simulink library "HighClearance_library"  (R2019b)
settings: Solver=VariableStepAuto  StartTime=0.0  StopTime=10.0  RelTol=1e-3
undefined symbols (not defined in the file): bangBang_maxOut, baseClearance, controlTolerance, controlWaitTime, ctrlWarningTime, currentControl_IC, currentControl_Ki, currentControl_Kp, currentControl_maxOut, currentControl_minOut, defaultPositionSensor_BrkPnts, DiscIntNeverNeededParam, errDelay, heightCalibrating_e, heightControlToleranceStart, heightControlToleranceStop, heightDiffTolerance, heightDown_e, heightError_e, heightMovingDown_e, heightMovingUp_e, heightTolerance, heightToleranceRoad, heightUnknown_e, heightUp_e, IOD_OK, legMovingTimeout, minDistanceMoving, movementTimeOut, noMovementTimeOut, plausiDistance, positionControl_IC, positionControl_Ki, positionControl_Kp, positionControl_maxOut, positionControl_minOut, positionSensor_tblData, sensorCutOffHz, step_time, trackWidthTolerance, useSensorFilter
libraries: $bdroot x29, simulink x1
settings Model: Creator=lemaya  LastModifiedBy=milesluc
settings DataIOCC: ReturnWorkspaceOutputs=off
settings DebuggingCC: ArithmeticOperatorsInVariantConditions=warning
settings SFSimCC: SimUseLocalCustomCode=off  CustomCodeUndefinedFunction=UseInterfaceOnly
settings RTWCC: RTWUseLocalCustomCode=off
settings CodeAppCC: StateflowObjectComments=on

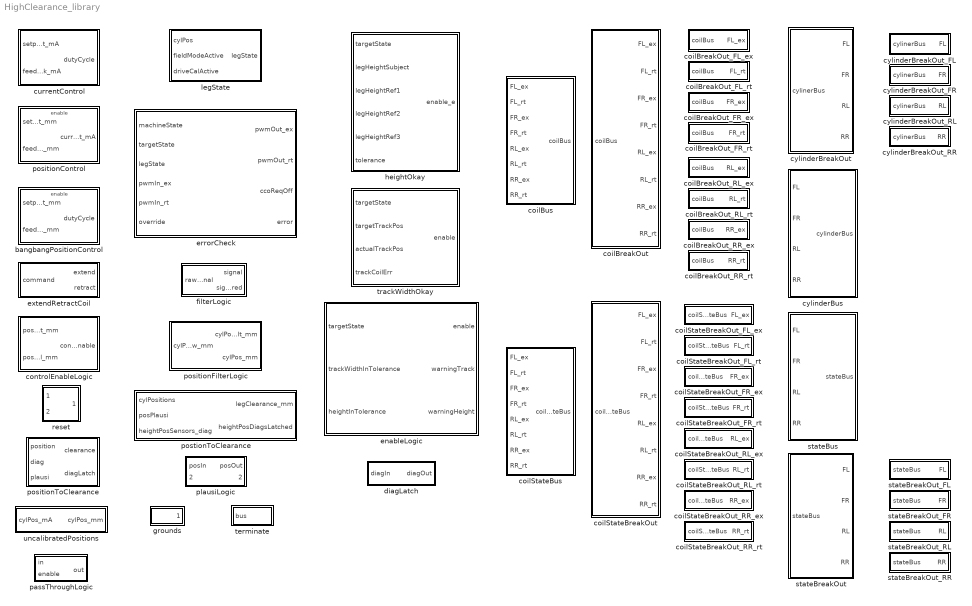
== system HighClearance_library ==
  bangbangPositionControl : Subsystem
  coilBreakOut : Subsystem
  coilBreakOut_FL_ex : Subsystem
  coilBreakOut_FL_rt : Subsystem
  coilBreakOut_FR_ex : Subsystem
  coilBreakOut_FR_rt : Subsystem
  coilBreakOut_RL_ex : Subsystem
  coilBreakOut_RL_rt : Subsystem
  coilBreakOut_RR_ex : Subsystem
  coilBreakOut_RR_rt : Subsystem
  coilBus : Subsystem
  coilStateBreakOut : Subsystem
  coilStateBreakOut_FL_ex : Subsystem
  coilStateBreakOut_FL_rt : Subsystem
  coilStateBreakOut_FR_ex : Subsystem
  coilStateBreakOut_FR_rt : Subsystem
  coilStateBreakOut_RL_ex : Subsystem
  coilStateBreakOut_RL_rt : Subsystem
  coilStateBreakOut_RR_ex : Subsystem
  coilStateBreakOut_RR_rt : Subsystem
  coilStateBus : Subsystem
  controlEnableLogic : Subsystem
  currentControl : Subsystem
  cylinderBreakOut : Subsystem
  cylinderBreakOut_FL : Subsystem
  cylinderBreakOut_FR : Subsystem
  cylinderBreakOut_RL : Subsystem
  cylinderBreakOut_RR : Subsystem
  cylinderBus : Subsystem
  diagLatch : Stateflow chart  TreatAsAtomicUnit=on
  enableLogic : Stateflow chart  TreatAsAtomicUnit=on
  errorCheck : Stateflow chart  TreatAsAtomicUnit=on
  extendRetractCoil : Subsystem
  filterLogic : Subsystem
  grounds : Subsystem
  heightOkay : Stateflow chart  TreatAsAtomicUnit=on
  legState : Stateflow chart  TreatAsAtomicUnit=on
  passThroughLogic : Subsystem
  plausiLogic : Subsystem
  positionControl : Subsystem
  positionFilterLogic : Subsystem
  positionToClearance : Subsystem
  postionToClearance : Subsystem
  reset : Subsystem
  stateBreakOut : Subsystem
  stateBreakOut_FL : Subsystem
  stateBreakOut_FR : Subsystem
  stateBreakOut_RL : Subsystem
  stateBreakOut_RR : Subsystem
  stateBus : Subsystem
  terminate : Subsystem
  trackWidthOkay : Stateflow chart  TreatAsAtomicUnit=on
  uncalibratedPositions : Subsystem

== system HighClearance_library/bangbangPositionControl ==
  setpoint_mm : Inport
  feedback_mm : Inport  Port=2
  Enable : EnablePort  StatesWhenEnabling=reset
  Sum : Sum  Inputs=|+-
  extendRetractLogic : Stateflow chart  TreatAsAtomicUnit=on
  dutyCycle : Outport  OutputWhenDisabled=reset  InitialOutput=[0]
  wires:
  extendRetractLogic/1(pwm) -> dutyCycle/1
  Sum/1 -> extendRetractLogic/1(error)
  feedback_mm/1 -> Sum/2
  setpoint_mm/1 -> Sum/1

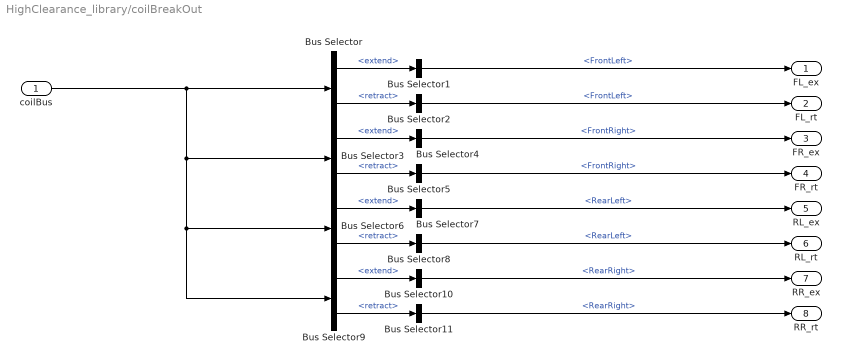
== system HighClearance_library/coilBreakOut ==
  coilBus : Inport  OutDataTypeStr=Bus: CoilBus
  Bus Selector{,3,6,9} (4 alike) : BusSelector  OutputSignals=extend,retract
  Bus Selector1 : BusSelector  OutputSignals=FrontLeft
  Bus Selector10 : BusSelector  OutputSignals=RearRight
  Bus Selector11 : BusSelector  OutputSignals=RearRight
  Bus Selector2 : BusSelector  OutputSignals=FrontLeft
  Bus Selector4 : BusSelector  OutputSignals=FrontRight
  Bus Selector5 : BusSelector  OutputSignals=FrontRight
  Bus Selector7 : BusSelector  OutputSignals=RearLeft
  Bus Selector8 : BusSelector  OutputSignals=RearLeft
  FL_ex : Outport
  FL_rt : Outport  Port=2
  FR_ex : Outport  Port=3
  FR_rt : Outport  Port=4
  RL_ex : Outport  Port=5
  RL_rt : Outport  Port=6
  RR_ex : Outport  Port=7
  RR_rt : Outport  Port=8
  wires:
  coilBus/1 -> Bus Selector/1, Bus Selector3/1, Bus Selector6/1, Bus Selector9/1
  Bus Selector9/2 -> Bus Selector11/1  "<retract>"
  Bus Selector11/1 -> RR_rt/1  "<RearRight>"
  Bus Selector10/1 -> RR_ex/1  "<RearRight>"
  Bus Selector9/1 -> Bus Selector10/1  "<extend>"
  Bus Selector6/2 -> Bus Selector8/1  "<retract>"
  Bus Selector8/1 -> RL_rt/1  "<RearLeft>"
  Bus Selector7/1 -> RL_ex/1  "<RearLeft>"
  Bus Selector6/1 -> Bus Selector7/1  "<extend>"
  Bus Selector3/2 -> Bus Selector5/1  "<retract>"
  Bus Selector5/1 -> FR_rt/1  "<FrontRight>"
  Bus Selector4/1 -> FR_ex/1  "<FrontRight>"
  Bus Selector3/1 -> Bus Selector4/1  "<extend>"
  Bus Selector/2 -> Bus Selector2/1  "<retract>"
  Bus Selector2/1 -> FL_rt/1  "<FrontLeft>"
  Bus Selector1/1 -> FL_ex/1  "<FrontLeft>"
  Bus Selector/1 -> Bus Selector1/1  "<extend>"

== system HighClearance_library/coilBreakOut_FL_ex ==
  coilBus : Inport  OutDataTypeStr=Bus: CoilBus
  Bus Selector : BusSelector  OutputSignals=extend
  Bus Selector1 : BusSelector  OutputSignals=FrontLeft
  FL_ex : Outport
  wires:
  Bus Selector/1 -> Bus Selector1/1  "<extend>"
  Bus Selector1/1 -> FL_ex/1  "<FrontLeft>"
  coilBus/1 -> Bus Selector/1

== system HighClearance_library/coilBreakOut_FL_rt ==
  coilBus : Inport  OutDataTypeStr=Bus: CoilBus
  Bus Selector : BusSelector  OutputSignals=retract
  Bus Selector1 : BusSelector  OutputSignals=FrontLeft
  FL_rt : Outport
  wires:
  coilBus/1 -> Bus Selector/1
  Bus Selector1/1 -> FL_rt/1  "<FrontLeft>"
  Bus Selector/1 -> Bus Selector1/1  "<retract>"

== system HighClearance_library/coilBreakOut_FR_ex ==
  coilBus : Inport  OutDataTypeStr=Bus: CoilBus
  Bus Selector : BusSelector  OutputSignals=extend
  Bus Selector1 : BusSelector  OutputSignals=FrontRight
  FR_ex : Outport
  wires:
  coilBus/1 -> Bus Selector/1
  Bus Selector1/1 -> FR_ex/1  "<FrontRight>"
  Bus Selector/1 -> Bus Selector1/1  "<extend>"

== system HighClearance_library/coilBreakOut_FR_rt ==
  coilBus : Inport  OutDataTypeStr=Bus: CoilBus
  Bus Selector : BusSelector  OutputSignals=retract
  Bus Selector1 : BusSelector  OutputSignals=FrontRight
  FR_rt : Outport
  wires:
  Bus Selector/1 -> Bus Selector1/1  "<retract>"
  Bus Selector1/1 -> FR_rt/1  "<FrontRight>"
  coilBus/1 -> Bus Selector/1

== system HighClearance_library/coilBreakOut_RL_ex ==
  coilBus : Inport  OutDataTypeStr=Bus: CoilBus
  Bus Selector : BusSelector  OutputSignals=extend
  Bus Selector1 : BusSelector  OutputSignals=RearLeft
  RL_ex : Outport
  wires:
  coilBus/1 -> Bus Selector/1
  Bus Selector1/1 -> RL_ex/1  "<RearLeft>"
  Bus Selector/1 -> Bus Selector1/1  "<extend>"

== system HighClearance_library/coilBreakOut_RL_rt ==
  coilBus : Inport  OutDataTypeStr=Bus: CoilBus
  Bus Selector : BusSelector  OutputSignals=retract
  Bus Selector1 : BusSelector  OutputSignals=RearLeft
  RL_rt : Outport
  wires:
  Bus Selector/1 -> Bus Selector1/1  "<retract>"
  Bus Selector1/1 -> RL_rt/1  "<RearLeft>"
  coilBus/1 -> Bus Selector/1

== system HighClearance_library/coilBreakOut_RR_ex ==
  coilBus : Inport  OutDataTypeStr=Bus: CoilBus
  Bus Selector : BusSelector  OutputSignals=extend
  Bus Selector1 : BusSelector  OutputSignals=RearRight
  RR_ex : Outport
  wires:
  Bus Selector/1 -> Bus Selector1/1  "<extend>"
  Bus Selector1/1 -> RR_ex/1  "<RearRight>"
  coilBus/1 -> Bus Selector/1

== system HighClearance_library/coilBreakOut_RR_rt ==
  coilBus : Inport  OutDataTypeStr=Bus: CoilBus
  Bus Selector : BusSelector  OutputSignals=retract
  Bus Selector1 : BusSelector  OutputSignals=RearRight
  RR_rt : Outport
  wires:
  coilBus/1 -> Bus Selector/1
  Bus Selector1/1 -> RR_rt/1  "<RearRight>"
  Bus Selector/1 -> Bus Selector1/1  "<retract>"

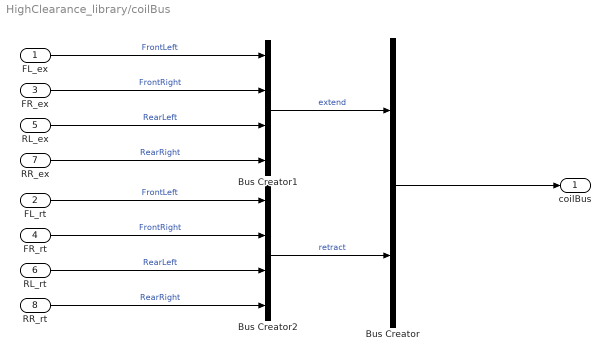
== system HighClearance_library/coilBus ==
  FL_ex : Inport
  FL_rt : Inport  Port=2
  FR_ex : Inport  Port=3
  FR_rt : Inport  Port=4
  RL_ex : Inport  Port=5
  RL_rt : Inport  Port=6
  RR_ex : Inport  Port=7
  RR_rt : Inport  Port=8
  Bus Creator : BusCreator  Inputs=2  OutDataTypeStr=Bus: CoilBus  NonVirtualBus=on
  Bus Creator1 : BusCreator  Inputs=4  OutDataTypeStr=Bus: CylinderBus  NonVirtualBus=on
  Bus Creator2 : BusCreator  Inputs=4  OutDataTypeStr=Bus: CylinderBus  NonVirtualBus=on
  coilBus : Outport  OutDataTypeStr=Bus: CoilBus
  wires:
  FL_ex/1 -> Bus Creator1/1  "FrontLeft"
  Bus Creator/1 -> coilBus/1
  FR_ex/1 -> Bus Creator1/2  "FrontRight"
  RL_ex/1 -> Bus Creator1/3  "RearLeft"
  RR_ex/1 -> Bus Creator1/4  "RearRight"
  Bus Creator1/1 -> Bus Creator/1  "extend"
  Bus Creator2/1 -> Bus Creator/2  "retract"
  FL_rt/1 -> Bus Creator2/1  "FrontLeft"
  FR_rt/1 -> Bus Creator2/2  "FrontRight"
  RL_rt/1 -> Bus Creator2/3  "RearLeft"
  RR_rt/1 -> Bus Creator2/4  "RearRight"

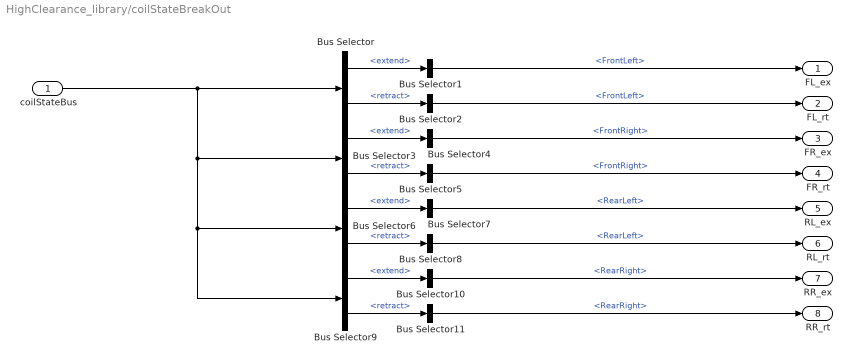
== system HighClearance_library/coilStateBreakOut ==
  coilStateBus : Inport  OutDataTypeStr=Bus: CoilStateBus
  Bus Selector{,3,6,9} (4 alike) : BusSelector  OutputSignals=extend,retract
  Bus Selector1 : BusSelector  OutputSignals=FrontLeft
  Bus Selector10 : BusSelector  OutputSignals=RearRight
  Bus Selector11 : BusSelector  OutputSignals=RearRight
  Bus Selector2 : BusSelector  OutputSignals=FrontLeft
  Bus Selector4 : BusSelector  OutputSignals=FrontRight
  Bus Selector5 : BusSelector  OutputSignals=FrontRight
  Bus Selector7 : BusSelector  OutputSignals=RearLeft
  Bus Selector8 : BusSelector  OutputSignals=RearLeft
  FL_ex : Outport
  FL_rt : Outport  Port=2
  FR_ex : Outport  Port=3
  FR_rt : Outport  Port=4
  RL_ex : Outport  Port=5
  RL_rt : Outport  Port=6
  RR_ex : Outport  Port=7
  RR_rt : Outport  Port=8
  wires:
  coilStateBus/1 -> Bus Selector/1, Bus Selector3/1, Bus Selector6/1, Bus Selector9/1
  Bus Selector9/2 -> Bus Selector11/1  "<retract>"
  Bus Selector11/1 -> RR_rt/1  "<RearRight>"
  Bus Selector10/1 -> RR_ex/1  "<RearRight>"
  Bus Selector9/1 -> Bus Selector10/1  "<extend>"
  Bus Selector6/2 -> Bus Selector8/1  "<retract>"
  Bus Selector8/1 -> RL_rt/1  "<RearLeft>"
  Bus Selector7/1 -> RL_ex/1  "<RearLeft>"
  Bus Selector6/1 -> Bus Selector7/1  "<extend>"
  Bus Selector3/2 -> Bus Selector5/1  "<retract>"
  Bus Selector5/1 -> FR_rt/1  "<FrontRight>"
  Bus Selector4/1 -> FR_ex/1  "<FrontRight>"
  Bus Selector3/1 -> Bus Selector4/1  "<extend>"
  Bus Selector/2 -> Bus Selector2/1  "<retract>"
  Bus Selector2/1 -> FL_rt/1  "<FrontLeft>"
  Bus Selector1/1 -> FL_ex/1  "<FrontLeft>"
  Bus Selector/1 -> Bus Selector1/1  "<extend>"

== system HighClearance_library/coilStateBreakOut_FL_ex ==
  coilStateBus : Inport  OutDataTypeStr=Bus: CoilStateBus
  Bus Selector : BusSelector  OutputSignals=extend
  Bus Selector1 : BusSelector  OutputSignals=FrontLeft
  FL_ex : Outport
  wires:
  Bus Selector/1 -> Bus Selector1/1  "<extend>"
  Bus Selector1/1 -> FL_ex/1  "<FrontLeft>"
  coilStateBus/1 -> Bus Selector/1

== system HighClearance_library/coilStateBreakOut_FL_rt ==
  coilStateBus : Inport  OutDataTypeStr=Bus: CoilStateBus
  Bus Selector : BusSelector  OutputSignals=retract
  Bus Selector1 : BusSelector  OutputSignals=FrontLeft
  FL_rt : Outport
  wires:
  coilStateBus/1 -> Bus Selector/1
  Bus Selector1/1 -> FL_rt/1  "<FrontLeft>"
  Bus Selector/1 -> Bus Selector1/1  "<retract>"

== system HighClearance_library/coilStateBreakOut_FR_ex ==
  coilStateBus : Inport  OutDataTypeStr=Bus: CoilStateBus
  Bus Selector : BusSelector  OutputSignals=extend
  Bus Selector1 : BusSelector  OutputSignals=FrontRight
  FR_ex : Outport
  wires:
  coilStateBus/1 -> Bus Selector/1
  Bus Selector1/1 -> FR_ex/1  "<FrontRight>"
  Bus Selector/1 -> Bus Selector1/1  "<extend>"

== system HighClearance_library/coilStateBreakOut_FR_rt ==
  coilStateBus : Inport  OutDataTypeStr=Bus: CoilStateBus
  Bus Selector : BusSelector  OutputSignals=retract
  Bus Selector1 : BusSelector  OutputSignals=FrontRight
  FR_rt : Outport
  wires:
  Bus Selector/1 -> Bus Selector1/1  "<retract>"
  Bus Selector1/1 -> FR_rt/1  "<FrontRight>"
  coilStateBus/1 -> Bus Selector/1

== system HighClearance_library/coilStateBreakOut_RL_ex ==
  coilStateBus : Inport  OutDataTypeStr=Bus: CoilStateBus
  Bus Selector : BusSelector  OutputSignals=extend
  Bus Selector1 : BusSelector  OutputSignals=RearLeft
  RL_ex : Outport
  wires:
  coilStateBus/1 -> Bus Selector/1
  Bus Selector1/1 -> RL_ex/1  "<RearLeft>"
  Bus Selector/1 -> Bus Selector1/1  "<extend>"

== system HighClearance_library/coilStateBreakOut_RL_rt ==
  coilStateBus : Inport  OutDataTypeStr=Bus: CoilStateBus
  Bus Selector : BusSelector  OutputSignals=retract
  Bus Selector1 : BusSelector  OutputSignals=RearLeft
  RL_rt : Outport
  wires:
  Bus Selector/1 -> Bus Selector1/1  "<retract>"
  Bus Selector1/1 -> RL_rt/1  "<RearLeft>"
  coilStateBus/1 -> Bus Selector/1

== system HighClearance_library/coilStateBreakOut_RR_ex ==
  coilStateBus : Inport  OutDataTypeStr=Bus: CoilStateBus
  Bus Selector : BusSelector  OutputSignals=extend
  Bus Selector1 : BusSelector  OutputSignals=RearRight
  RR_ex : Outport
  wires:
  Bus Selector/1 -> Bus Selector1/1  "<extend>"
  Bus Selector1/1 -> RR_ex/1  "<RearRight>"
  coilStateBus/1 -> Bus Selector/1

== system HighClearance_library/coilStateBreakOut_RR_rt ==
  coilStateBus : Inport  OutDataTypeStr=Bus: CoilStateBus
  Bus Selector : BusSelector  OutputSignals=retract
  Bus Selector1 : BusSelector  OutputSignals=RearRight
  RR_rt : Outport
  wires:
  coilStateBus/1 -> Bus Selector/1
  Bus Selector1/1 -> RR_rt/1  "<RearRight>"
  Bus Selector/1 -> Bus Selector1/1  "<retract>"

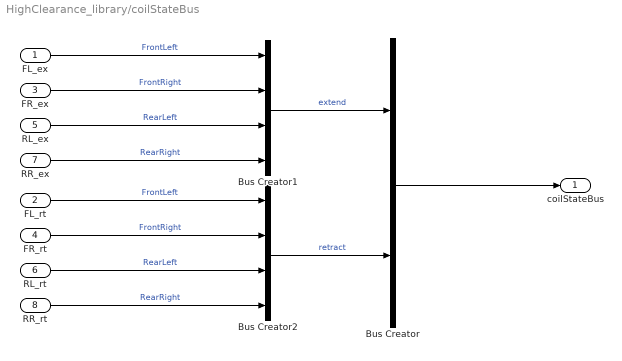
== system HighClearance_library/coilStateBus ==
  FL_ex : Inport
  FL_rt : Inport  Port=2
  FR_ex : Inport  Port=3
  FR_rt : Inport  Port=4
  RL_ex : Inport  Port=5
  RL_rt : Inport  Port=6
  RR_ex : Inport  Port=7
  RR_rt : Inport  Port=8
  Bus Creator : BusCreator  Inputs=2  OutDataTypeStr=Bus: CoilStateBus
  Bus Creator1 : BusCreator  Inputs=4  OutDataTypeStr=Bus: StateBus
  Bus Creator2 : BusCreator  Inputs=4  OutDataTypeStr=Bus: StateBus
  coilStateBus : Outport  OutDataTypeStr=Bus: CoilStateBus
  wires:
  FL_ex/1 -> Bus Creator1/1  "FrontLeft"
  Bus Creator/1 -> coilStateBus/1
  FR_ex/1 -> Bus Creator1/2  "FrontRight"
  RL_ex/1 -> Bus Creator1/3  "RearLeft"
  RR_ex/1 -> Bus Creator1/4  "RearRight"
  Bus Creator1/1 -> Bus Creator/1  "extend"
  Bus Creator2/1 -> Bus Creator/2  "retract"
  FL_rt/1 -> Bus Creator2/1  "FrontLeft"
  FR_rt/1 -> Bus Creator2/2  "FrontRight"
  RL_rt/1 -> Bus Creator2/3  "RearLeft"
  RR_rt/1 -> Bus Creator2/4  "RearRight"

== system HighClearance_library/controlEnableLogic ==
  postionTarget_mm : Inport
  positionActual_mm : Inport  Port=2
  enableLogic : Stateflow chart  TreatAsAtomicUnit=on
  controlEnable : Outport
  wires:
  postionTarget_mm/1 -> enableLogic/1(target)
  positionActual_mm/1 -> enableLogic/2(position)
  enableLogic/1(enable) -> controlEnable/1

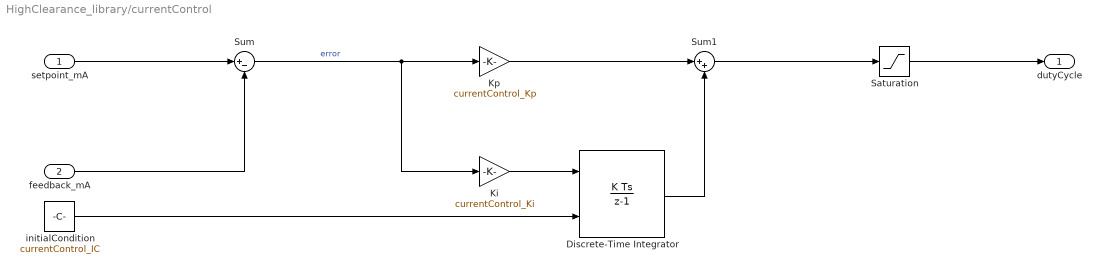
== system HighClearance_library/currentControl ==
  setpoint_mA : Inport
  feedback_mA : Inport  Port=2
  Discrete-Time Integrator : DiscreteIntegrator  InitialConditionSource=external  SampleTime=step_time  LimitOutput=on  UpperSaturationLimit=currentControl_maxOut  LowerSaturationLimit=currentControl_minOut  ICPrevOutput=DiscIntNeverNeededParam  ICPrevScaledInput=DiscIntNeverNeededParam
  Ki : Gain  Gain=currentControl_Ki
  Kp : Gain  Gain=currentControl_Kp
  Saturation : Saturate  UpperLimit=currentControl_maxOut  LowerLimit=currentControl_minOut
  Sum : Sum  Inputs=|+-
  Sum1 : Sum  Inputs=|++
  initialCondition : Constant  Value=currentControl_IC
  dutyCycle : Outport
  wires:
  Saturation/1 -> dutyCycle/1
  initialCondition/1 -> Discrete-Time Integrator/2
  Sum1/1 -> Saturation/1
  Discrete-Time Integrator/1 -> Sum1/2
  Ki/1 -> Discrete-Time Integrator/1
  Kp/1 -> Sum1/1
  Sum/1 -> Kp/1, Ki/1  "error"
  feedback_mA/1 -> Sum/2
  setpoint_mA/1 -> Sum/1

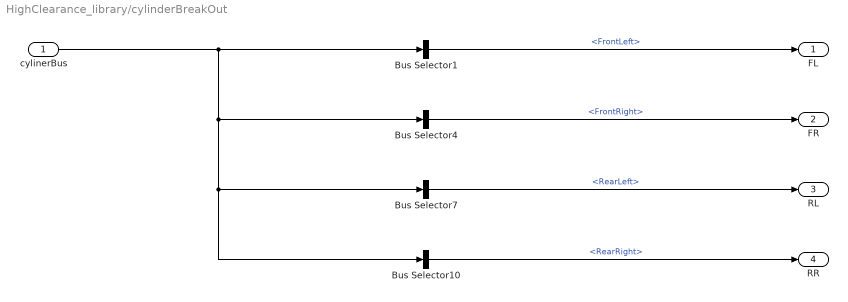
== system HighClearance_library/cylinderBreakOut ==
  cylinerBus : Inport  OutDataTypeStr=Bus: CylinderBus
  Bus Selector1 : BusSelector  OutputSignals=FrontLeft
  Bus Selector10 : BusSelector  OutputSignals=RearRight
  Bus Selector4 : BusSelector  OutputSignals=FrontRight
  Bus Selector7 : BusSelector  OutputSignals=RearLeft
  FL : Outport
  FR : Outport  Port=2
  RL : Outport  Port=3
  RR : Outport  Port=4
  wires:
  cylinerBus/1 -> Bus Selector1/1, Bus Selector4/1, Bus Selector7/1, Bus Selector10/1
  Bus Selector10/1 -> RR/1  "<RearRight>"
  Bus Selector7/1 -> RL/1  "<RearLeft>"
  Bus Selector4/1 -> FR/1  "<FrontRight>"
  Bus Selector1/1 -> FL/1  "<FrontLeft>"

== system HighClearance_library/cylinderBreakOut_FL ==
  cylinerBus : Inport  OutDataTypeStr=Bus: CylinderBus
  Bus Selector1 : BusSelector  OutputSignals=FrontLeft
  FL : Outport
  wires:
  cylinerBus/1 -> Bus Selector1/1
  Bus Selector1/1 -> FL/1  "<FrontLeft>"

== system HighClearance_library/cylinderBreakOut_FR ==
  cylinerBus : Inport  OutDataTypeStr=Bus: CylinderBus
  Bus Selector4 : BusSelector  OutputSignals=FrontRight
  FR : Outport
  wires:
  Bus Selector4/1 -> FR/1  "<FrontRight>"
  cylinerBus/1 -> Bus Selector4/1

== system HighClearance_library/cylinderBreakOut_RL ==
  cylinerBus : Inport  OutDataTypeStr=Bus: CylinderBus
  Bus Selector7 : BusSelector  OutputSignals=RearLeft
  RL : Outport
  wires:
  cylinerBus/1 -> Bus Selector7/1
  Bus Selector7/1 -> RL/1  "<RearLeft>"

== system HighClearance_library/cylinderBreakOut_RR ==
  cylinerBus : Inport  OutDataTypeStr=Bus: CylinderBus
  Bus Selector10 : BusSelector  OutputSignals=RearRight
  RR : Outport
  wires:
  Bus Selector10/1 -> RR/1  "<RearRight>"
  cylinerBus/1 -> Bus Selector10/1

== system HighClearance_library/cylinderBus ==
  FL : Inport
  FR : Inport  Port=2
  RL : Inport  Port=3
  RR : Inport  Port=4
  Bus Creator1 : BusCreator  Inputs=4  OutDataTypeStr=Bus: CylinderBus
  cylinderBus : Outport  OutDataTypeStr=Bus: CylinderBus
  wires:
  Bus Creator1/1 -> cylinderBus/1
  FL/1 -> Bus Creator1/1  "FrontLeft"
  FR/1 -> Bus Creator1/2  "FrontRight"
  RL/1 -> Bus Creator1/3  "RearLeft"
  RR/1 -> Bus Creator1/4  "RearRight"

== system HighClearance_library/extendRetractCoil ==
  command : Inport
  Abs : Abs
  Constant : Constant  Value=0  OutDataTypeStr=Inherit: Inherit via back propagation
  Switch : Switch  Criteria=u2 > Threshold
  Switch1 : Switch
  extend : Outport
  retract : Outport  Port=2
  wires:
  Abs/1 -> retract/1
  Switch1/1 -> Abs/1
  Constant/1 -> Switch/3, Switch1/1
  Switch/1 -> extend/1
  command/1 -> Switch1/2, Switch1/3, Switch/2, Switch/1

== system HighClearance_library/filterLogic ==
  rawSignal : Inport
  Switch : Switch  Criteria=u2 ~= 0
  cutoffFreq : Constant  Value=sensorCutOffHz
  filter : Subsystem  mask(Discrete Lowpass Filter){delta_t=step_time}
      mask prompts: delta_t "Sample time:"
      mask help: Discrete LPF filters the signal by the cutoff fequency
  rawSignal1 : InportShadow
  useSensorFilter : Constant  Value=useSensorFilter
  signal : Outport
  signalFiltered : Outport  Port=2
  wires:
  rawSignal1/1 -> Switch/3
  Switch/1 -> signal/1
  useSensorFilter/1 -> Switch/2
  cutoffFreq/1 -> filter/3(Cutoff_Hz)  "hz"
  rawSignal/1 -> filter/1(Signal), filter/2(IC)
  filter/1(filteredSignal) -> Switch/1, signalFiltered/1

== system HighClearance_library/grounds ==
  Data Type Conversion{,1..3} (4 alike) : DataTypeConversion  OutDataTypeStr=uint8
  Ground : Ground
  stateBus : $bdroot/stateBus
  gndBus : Outport
  wires:
  Ground/1 -> Data Type Conversion/1, Data Type Conversion1/1, Data Type Conversion2/1, Data Type Conversion3/1
  Data Type Conversion3/1 -> stateBus/4
  Data Type Conversion2/1 -> stateBus/3
  Data Type Conversion1/1 -> stateBus/2
  Data Type Conversion/1 -> stateBus/1
  stateBus/1 -> gndBus/1

== system HighClearance_library/passThroughLogic ==
  in : Inport
  enable : Inport  Port=2
  Data Type Conversion1 : DataTypeConversion
  Switch1 : Switch  Criteria=u2 > Threshold
  out : Outport
  wires:
  enable/1 -> Data Type Conversion1/1, Switch1/2
  Switch1/1 -> out/1
  in/1 -> Switch1/1
  Data Type Conversion1/1 -> Switch1/3

== system HighClearance_library/plausiLogic ==
  posIn : Inport
  enablePlausiCheck : Inport  Port=2
  Delay : Delay  DelayLength=3  SampleTime=step_time
  plausiCheck : Stateflow chart  TreatAsAtomicUnit=on
  posOut : Outport
  plausiErr : Outport  Port=2
  wires:
  enablePlausiCheck/1 -> plausiCheck/3(enableCheck)
  plausiCheck/2(plausiErr) -> plausiErr/1
  plausiCheck/1(positionOut) -> posOut/1
  posIn/1 -> plausiCheck/1(positionIn), Delay/1
  Delay/1 -> plausiCheck/2(positionDelay)

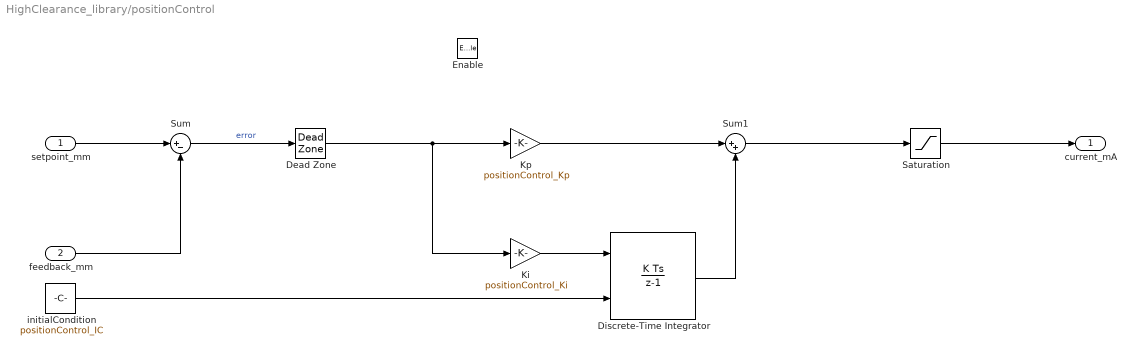
== system HighClearance_library/positionControl ==
  setpoint_mm : Inport
  feedback_mm : Inport  Port=2
  Enable : EnablePort  StatesWhenEnabling=reset
  Dead Zone : DeadZone  LowerValue=-controlTolerance  UpperValue=controlTolerance  SaturateOnIntegerOverflow=on
  Discrete-Time Integrator : DiscreteIntegrator  gainval=1  InitialConditionSource=external  SampleTime=step_time  LimitOutput=on  UpperSaturationLimit=positionControl_maxOut  LowerSaturationLimit=positionControl_minOut  ICPrevOutput=DiscIntNeverNeededParam  ICPrevScaledInput=DiscIntNeverNeededParam
  Ki : Gain  Gain=positionControl_Ki
  Kp : Gain  Gain=positionControl_Kp
  Saturation : Saturate  UpperLimit=positionControl_maxOut  LowerLimit=positionControl_minOut
  Sum : Sum  Inputs=|+-
  Sum1 : Sum  Inputs=|++
  initialCondition : Constant  Value=positionControl_IC
  current_mA : Outport
  wires:
  setpoint_mm/1 -> Sum/1
  Saturation/1 -> current_mA/1
  initialCondition/1 -> Discrete-Time Integrator/2
  Sum1/1 -> Saturation/1
  Discrete-Time Integrator/1 -> Sum1/2
  Ki/1 -> Discrete-Time Integrator/1
  Kp/1 -> Sum1/1
  Sum/1 -> Dead Zone/1  "error"
  feedback_mm/1 -> Sum/2
  Dead Zone/1 -> Kp/1, Ki/1

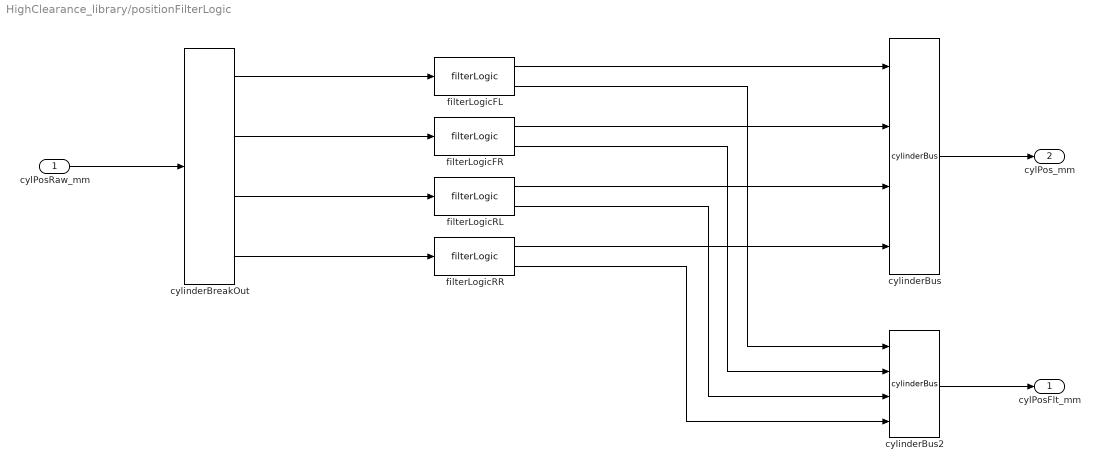
== system HighClearance_library/positionFilterLogic ==
  cylPosRaw_mm : Inport
  cylinderBreakOut : $bdroot/cylinderBreakOut
  cylinderBus : $bdroot/cylinderBus
  cylinderBus2 : $bdroot/cylinderBus
  filterLogicFL : $bdroot/filterLogic
  filterLogicFR : $bdroot/filterLogic
  filterLogicRL : $bdroot/filterLogic
  filterLogicRR : $bdroot/filterLogic
  cylPosFlt_mm : Outport
  cylPos_mm : Outport  Port=2
  wires:
  cylinderBreakOut/4 -> filterLogicRR/1
  cylinderBreakOut/3 -> filterLogicRL/1
  cylinderBreakOut/2 -> filterLogicFR/1
  cylinderBreakOut/1 -> filterLogicFL/1
  cylPosRaw_mm/1 -> cylinderBreakOut/1
  cylinderBus/1 -> cylPos_mm/1
  filterLogicFL/1 -> cylinderBus/1
  filterLogicFR/1 -> cylinderBus/2
  filterLogicRL/1 -> cylinderBus/3
  filterLogicRR/1 -> cylinderBus/4
  cylinderBus2/1 -> cylPosFlt_mm/1
  filterLogicFL/2 -> cylinderBus2/1
  filterLogicFR/2 -> cylinderBus2/2
  filterLogicRL/2 -> cylinderBus2/3
  filterLogicRR/2 -> cylinderBus2/4

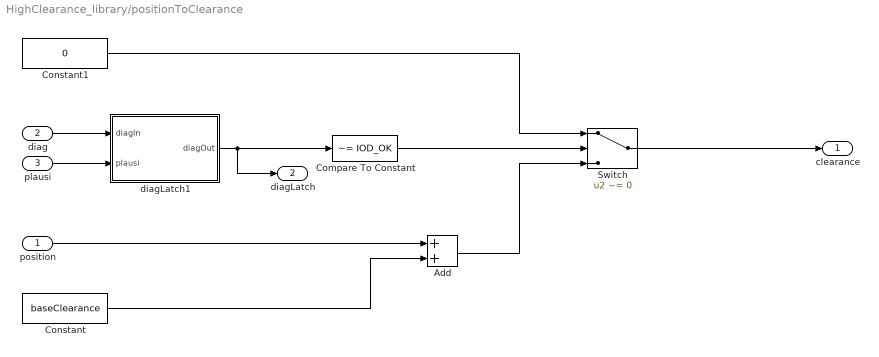
== system HighClearance_library/positionToClearance ==
  position : Inport
  diag : Inport  Port=2
  plausi : Inport  Port=3
  Add : Sum
  Compare To Constant : simulink/Logic and Bit Operations/Compare To Constant  relop=~=  const=IOD_OK  OutDataTypeStr=boolean
  Constant : Constant  Value=baseClearance
  Constant1 : Constant  Value=0  OutDataTypeStr=Inherit: Inherit via back propagation
  Switch : Switch  Criteria=u2 ~= 0
  diagLatch1 : Stateflow chart  TreatAsAtomicUnit=on
  clearance : Outport
  diagLatch : Outport  Port=2
  wires:
  plausi/1 -> diagLatch1/2(plausi)
  Compare To Constant/1 -> Switch/2
  diagLatch1/1(diagOut) -> Compare To Constant/1, diagLatch/1
  Add/1 -> Switch/3
  Constant1/1 -> Switch/1
  diag/1 -> diagLatch1/1(diagIn)
  Switch/1 -> clearance/1
  Constant/1 -> Add/2
  position/1 -> Add/1

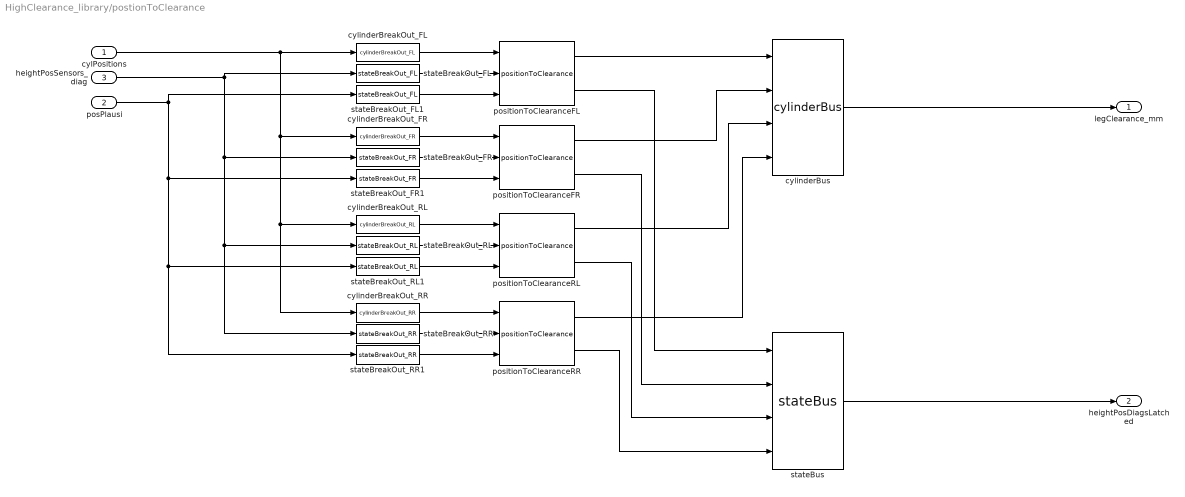
== system HighClearance_library/postionToClearance ==
  cylPositions : Inport  OutDataTypeStr=Bus: CylinderBus
  posPlausi : Inport  Port=2  OutDataTypeStr=Bus: StateBus
  heightPosSensors_diag : Inport  Port=3  OutDataTypeStr=Bus: StateBus
  cylinderBreakOut_FL : $bdroot/cylinderBreakOut_FL
  cylinderBreakOut_FR : $bdroot/cylinderBreakOut_FR
  cylinderBreakOut_RL : $bdroot/cylinderBreakOut_RL
  cylinderBreakOut_RR : $bdroot/cylinderBreakOut_RR
  cylinderBus : $bdroot/cylinderBus
  positionToClearanceFL : $bdroot/positionToClearance
  positionToClearanceFR : $bdroot/positionToClearance
  positionToClearanceRL : $bdroot/positionToClearance
  positionToClearanceRR : $bdroot/positionToClearance
  stateBreakOut_FL : $bdroot/stateBreakOut_FL
  stateBreakOut_FL1 : $bdroot/stateBreakOut_FL
  stateBreakOut_FR : $bdroot/stateBreakOut_FR
  stateBreakOut_FR1 : $bdroot/stateBreakOut_FR
  stateBreakOut_RL : $bdroot/stateBreakOut_RL
  stateBreakOut_RL1 : $bdroot/stateBreakOut_RL
  stateBreakOut_RR : $bdroot/stateBreakOut_RR
  stateBreakOut_RR1 : $bdroot/stateBreakOut_RR
  stateBus : $bdroot/stateBus
  legClearance_mm : Outport  OutDataTypeStr=Bus: CylinderBus
  heightPosDiagsLatched : Outport  Port=2  OutDataTypeStr=Bus: StateBus
  wires:
  stateBreakOut_RR1/1 -> positionToClearanceRR/3
  stateBreakOut_RL1/1 -> positionToClearanceRL/3
  stateBreakOut_FR1/1 -> positionToClearanceFR/3
  stateBreakOut_FL1/1 -> positionToClearanceFL/3
  posPlausi/1 -> stateBreakOut_FR1/1, stateBreakOut_RL1/1, stateBreakOut_RR1/1, stateBreakOut_FL1/1
  positionToClearanceFL/2 -> stateBus/1
  positionToClearanceFR/2 -> stateBus/2
  positionToClearanceRL/2 -> stateBus/3
  positionToClearanceRR/2 -> stateBus/4
  stateBus/1 -> heightPosDiagsLatched/1
  heightPosSensors_diag/1 -> stateBreakOut_FR/1, stateBreakOut_RL/1, stateBreakOut_RR/1, stateBreakOut_FL/1
  cylPositions/1 -> cylinderBreakOut_FL/1, cylinderBreakOut_FR/1, cylinderBreakOut_RL/1, cylinderBreakOut_RR/1
  cylinderBus/1 -> legClearance_mm/1
  positionToClearanceFL/1 -> cylinderBus/1
  positionToClearanceRR/1 -> cylinderBus/4
  positionToClearanceFR/1 -> cylinderBus/2
  positionToClearanceRL/1 -> cylinderBus/3
  cylinderBreakOut_RR/1 -> positionToClearanceRR/1
  cylinderBreakOut_RL/1 -> positionToClearanceRL/1
  cylinderBreakOut_FR/1 -> positionToClearanceFR/1
  cylinderBreakOut_FL/1 -> positionToClearanceFL/1
  stateBreakOut_RR/1 -> positionToClearanceRR/2
  stateBreakOut_RL/1 -> positionToClearanceRL/2
  stateBreakOut_FR/1 -> positionToClearanceFR/2
  stateBreakOut_FL/1 -> positionToClearanceFL/2

== system HighClearance_library/reset ==
  enable : Inport
  signalIn : Inport  Port=2
  Switch : Switch  Criteria=u2 > Threshold
  signalOut : Outport
  wires:
  Switch/1 -> signalOut/1
  signalIn/1 -> Switch/1
  enable/1 -> Switch/2, Switch/3

== system HighClearance_library/stateBreakOut ==
  stateBus : Inport  OutDataTypeStr=Bus: StateBus
  Bus Selector1 : BusSelector  OutputSignals=FrontLeft
  Bus Selector10 : BusSelector  OutputSignals=RearRight
  Bus Selector4 : BusSelector  OutputSignals=FrontRight
  Bus Selector7 : BusSelector  OutputSignals=RearLeft
  FL : Outport
  FR : Outport  Port=2
  RL : Outport  Port=3
  RR : Outport  Port=4
  wires:
  stateBus/1 -> Bus Selector1/1, Bus Selector4/1, Bus Selector7/1, Bus Selector10/1
  Bus Selector10/1 -> RR/1  "<RearRight>"
  Bus Selector7/1 -> RL/1  "<RearLeft>"
  Bus Selector4/1 -> FR/1  "<FrontRight>"
  Bus Selector1/1 -> FL/1  "<FrontLeft>"

== system HighClearance_library/stateBreakOut_FL ==
  stateBus : Inport  OutDataTypeStr=Bus: StateBus
  Bus Selector1 : BusSelector  OutputSignals=FrontLeft
  FL : Outport
  wires:
  stateBus/1 -> Bus Selector1/1
  Bus Selector1/1 -> FL/1  "<FrontLeft>"

== system HighClearance_library/stateBreakOut_FR ==
  stateBus : Inport  OutDataTypeStr=Bus: StateBus
  Bus Selector1 : BusSelector  OutputSignals=FrontRight
  FR : Outport
  wires:
  Bus Selector1/1 -> FR/1  "<FrontRight>"
  stateBus/1 -> Bus Selector1/1

== system HighClearance_library/stateBreakOut_RL ==
  stateBus : Inport  OutDataTypeStr=Bus: StateBus
  Bus Selector1 : BusSelector  OutputSignals=RearLeft
  RL : Outport
  wires:
  stateBus/1 -> Bus Selector1/1
  Bus Selector1/1 -> RL/1  "<RearLeft>"

== system HighClearance_library/stateBreakOut_RR ==
  stateBus : Inport  OutDataTypeStr=Bus: StateBus
  Bus Selector1 : BusSelector  OutputSignals=RearRight
  RR : Outport
  wires:
  Bus Selector1/1 -> RR/1  "<RearRight>"
  stateBus/1 -> Bus Selector1/1

== system HighClearance_library/stateBus ==
  FL : Inport
  FR : Inport  Port=2
  RL : Inport  Port=3
  RR : Inport  Port=4
  Bus Creator1 : BusCreator  Inputs=4  OutDataTypeStr=Bus: StateBus
  stateBus : Outport  OutDataTypeStr=Bus: StateBus
  wires:
  RR/1 -> Bus Creator1/4  "RearRight"
  RL/1 -> Bus Creator1/3  "RearLeft"
  FR/1 -> Bus Creator1/2  "FrontRight"
  FL/1 -> Bus Creator1/1  "FrontLeft"
  Bus Creator1/1 -> stateBus/1

== system HighClearance_library/terminate ==
  bus : Inport
  Terminator{,1..3} (4 alike) : Terminator
  cylinderBreakOut1 : $bdroot/cylinderBreakOut
  wires:
  cylinderBreakOut1/2 -> Terminator1/1
  cylinderBreakOut1/1 -> Terminator/1
  cylinderBreakOut1/3 -> Terminator2/1
  bus/1 -> cylinderBreakOut1/1
  cylinderBreakOut1/4 -> Terminator3/1

== system HighClearance_library/uncalibratedPositions ==
  cylPos_mA : Inport
  1-D Lookup Table{,1..3} (4 alike) : Lookup_n-D  NumberOfTableDimensions=1  BreakpointsForDimension1=defaultPositionSensor_BrkPnts  Table=positionSensor_tblData  ExtrapMethod=Clip  UseLastTableValue=on  InternalRulePriority=Speed  RndMeth=Simplest  InputSameDT=on
  cylinderBreakOut : $bdroot/cylinderBreakOut
  cylinderBus : $bdroot/cylinderBus
  cylPos_mm : Outport
  wires:
  cylPos_mA/1 -> cylinderBreakOut/1
  cylinderBreakOut/1 -> 1-D Lookup Table/1
  cylinderBreakOut/2 -> 1-D Lookup Table1/1
  cylinderBreakOut/3 -> 1-D Lookup Table2/1
  cylinderBreakOut/4 -> 1-D Lookup Table3/1
  1-D Lookup Table/1 -> cylinderBus/1
  1-D Lookup Table1/1 -> cylinderBus/2
  1-D Lookup Table2/1 -> cylinderBus/3
  1-D Lookup Table3/1 -> cylinderBus/4
  cylinderBus/1 -> cylPos_mm/1

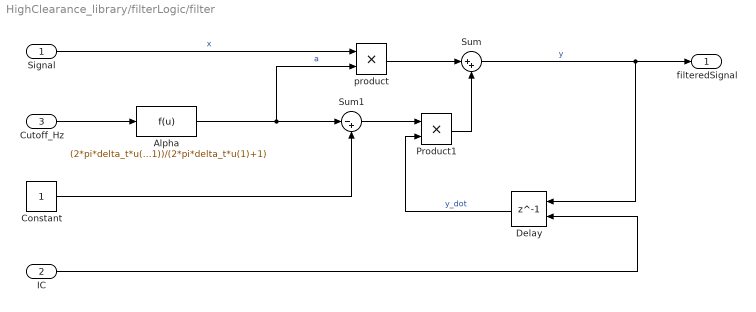
== system HighClearance_library/filterLogic/filter ==
  Signal : Inport
  IC : Inport  Port=2
  Cutoff_Hz : Inport  Port=3
  Alpha : Fcn  Expr=(2*pi*delta_t*u(1))/(2*pi*delta_t*u(1)+1)  SampleTime=delta_t
  Constant : Constant  OutDataTypeStr=single
  Delay : Delay  DelayLength=1  InitialConditionSource=Input port  InitialCondition=0
      settings: InputPortMap=u0,p4
  Product1 : Product
  Sum : Sum  Inputs=|++
  Sum1 : Sum  Inputs=|-+
  product : Product
  filteredSignal : Outport
  wires:
  IC/1 -> Delay/2
  Cutoff_Hz/1 -> Alpha/1
  Signal/1 -> product/1  "x"
  Alpha/1 -> Sum1/1, product/2  "a"
  product/1 -> Sum/1
  Sum/1 -> Delay/1, filteredSignal/1  "y"
  Constant/1 -> Sum1/2
  Sum1/1 -> Product1/1
  Delay/1 -> Product1/2  "y_dot"
  Product1/1 -> Sum/2

== stateflow chart HighClearance_library/controlEnableLogic/enableLogic ==
  state out = error [function]
    (default) -> (junction 17) : { out = abs(target-position) }
  state stopped
    en: enable = 0;
  state moving
    en: enable = 1;
    state outOfTolerance
    state inTolerance
    (default) -> outOfTolerance
    outOfTolerance -> inTolerance : [error() <= controlTolerance]
    inTolerance -> outOfTolerance [order 2] : [error() > controlTolerance]
  (default) -> stopped
  stopped -> moving : [hasChanged(target)]
  moving -> moving : [hasChanged(target)]
  inTolerance -> stopped [order 1] : after(controlWaitTime,msec)
  data: out function_output double; target input; position input; enable output; controlTolerance parameter; controlWaitTime parameter

== stateflow chart HighClearance_library/legState ==
  state normalOperaion
    state stopped
      en: prevPos = cylPos;
      state Up
        en: legState = heightUp_e;
      state Down
        en: legState = heightDown_e;
      state Unknown
        en: legState = heightUnknown_e;
    state moving
      en: prevPos = cylPos;
      state movingUp
        en: legState = heightMovingUp_e;
      state movingDown
        en: legState = heightMovingDown_e;
    (default) -> (junction 55) [order 1]
    (junction 645) -> (junction 55)
    (junction 55) -> Up [order 1] : [checkUpOrDown(cylPos) == heightUp_e ]
    (junction 88) -> movingUp : [(cylPos - prevPos) >= minDistanceMoving]
    (junction 98) -> (junction 645)
    (junction 55) -> (junction 56) [order 2]
    (junction 89) -> (junction 88) [order 2]
    (junction 56) -> Down : [checkUpOrDown(cylPos) == heightDown_e ]
    stopped -> (junction 641) : [checkUpOrDown(cylPos) != heightUp_e]
    (junction 641) -> (junction 89) : [checkUpOrDown(cylPos) != heightDown_e]
    (junction 89) -> movingDown [order 1] : [(prevPos - cylPos) >= minDistanceMoving]
    (junction 94) -> (junction 89)
    moving -> (junction 94) [order 2]
    (default) -> Unknown [order 2]
    moving -> Unknown [order 3] : after(legMovingTimeout,msec)
    Unknown -> (junction 648)
    moving -> (junction 78) [order 1]
    (junction 648) -> (junction 98)
    (junction 78) -> (junction 648)
  state error
    en: legState = heightError_e;
  (default) -> normalOperaion
  error -> normalOperaion : [cylPos > 0]
  normalOperaion -> error : [cylPos <= 0]
  data: legPos function_input single; state function_output uint8; tolerance local single; heightDown_e parameter; heightUp_e parameter; heightMovingUp_e parameter; heightMovingDown_e parameter; heightCalibrating_e parameter; heightError_e parameter; heightUnknown_e parameter; legState output uint8; positionSensor_tblData parameter; minDistanceMoving parameter; cylPos input; legMovingTimeout parameter; prevPos local single; heightTolerance parameter; baseClearance parameter; fieldModeActive input boolean; driveCalActive input boolean; heightToleranceRoad parameter
  function state = checkUpOrDown(legPos):
    | function state = checkUpOrDown(legPos)
    | 
    |     if( fieldModeActive || driveCalActive )
    |         tolerance = heightTolerance;
    |     else
    |         tolerance = heightToleranceRoad;
    |     end
    | 
    |     if( legPos >= ( positionSensor_tblData(2) + baseClearance - heightTolerance ))
    |         state = heightUp_e;
    |     elseif( legPos <= ( positionSensor_tblData(1) + baseClearance + tolerance ))
    |         state = heightDown_e;
    |     else
    |         state = heightUnknown_e;
    |     end
    | 
    | end

== stateflow chart HighClearance_library/positionToClearance/diagLatch1 ==
  state noError
    en: diagOut = IOD_OK;
  state plausiErr
    en: diagOut = 255;
  state IoErr
    en: diagOut = diagIn;
  (default) -> noError
  (junction 19) -> plausiErr : [plausi]
  (junction 14) -> (junction 19) [order 2]
  plausiErr -> IoErr : [diagIn]
  noError -> (junction 14) : after(errDelay,sec)
  (junction 14) -> IoErr [order 1] : [diagIn]
  data: diagIn input uint8; diagOut output uint8; errDelay parameter; IOD_OK parameter; plausi input

== stateflow chart HighClearance_library/diagLatch ==
  state noError
    en: diagOut = IOD_OK;
  state error
    en: diagOut = diagIn;
  (default) -> noError
  noError -> (junction 14) : after(errDelay,sec)
  (junction 14) -> error : [diagIn]
  data: diagIn input uint8; diagOut output uint8; errDelay parameter; IOD_OK parameter

== stateflow chart HighClearance_library/plausiLogic/plausiCheck ==
  state waitToCheck
    en:
    plausiErr = false;
    en,du:
    positionOut = positionIn;
    state disable
    state enable
    (default) -> disable
    disable -> enable : [enableCheck]
    enable -> disable [order 2] : [!enableCheck]
  state checking
    state plausiCheck
      en,du:
      positionOut = positionIn;
    state plausiError
      en:
      plausiErr = true;
      positionOut = positionDelay;
    plausiCheck -> plausiError : [abs(positionIn-positionDelay)>plausiDistance]
  (default) -> waitToCheck
  checking -> waitToCheck : [!enableCheck]
  enable -> plausiCheck [order 1] : after(errDelay,sec)
  data: positionOut output single; positionIn input single; plausiErr output uint8; errDelay parameter; positionDelay input; plausiDistance parameter; enableCheck input

== stateflow chart HighClearance_library/bangbangPositionControl/extendRetractLogic ==
  state extend
    en:
    pwm = bangBang_maxOut;
  state stop
    en: pwm = 0;
  state retract
    en:
    pwm = -bangBang_maxOut;
  (default) -> stop
  stop -> extend [order 1] : [error > heightControlToleranceStart]
  stop -> retract [order 2] : [error < -heightControlToleranceStart]
  extend -> stop : [error < heightControlToleranceStop]
  retract -> stop : [error > -heightControlToleranceStop]
  data: error input; pwm output; heightControlToleranceStart parameter; bangBang_maxOut parameter; heightUp_e parameter; heightMovingDown_e parameter; heightDown_e parameter; heightMovingUp_e parameter; heightError_e parameter; heightControlToleranceStop parameter

== stateflow chart HighClearance_library/errorCheck ==
  state errorChecking
    en: resetErrors(); pwmOut_ex = pwmIn_ex; pwmOut_rt = pwmIn_rt;
    du: pwmOut_ex = pwmIn_ex; pwmOut_rt = pwmIn_rt;
    state resetErrors [function]
      (default) -> (junction 163) : {error.movementErr1 = false;
          | error.movementErr2 = false;
          | error.noMovementErr = false;}
    state movmentError [parallel]
      settings: executionOrder=1
      state states
        state expectedToMove
          state stationary
          state moving
          (default) -> errorChecking.movmentError.states.expectedToMove.moving
          errorChecking.movmentError.states.expectedToMove.stationary -> errorChecking.movmentError.states.expectedToMove.moving [order 1] : [movingUpOrDown()]
          errorChecking.movmentError.states.expectedToMove.moving -> errorChecking.movmentError.states.expectedToMove.stationary : [!movingUpOrDown()]
        state notExpectedToMove
          state stationary
          state moving
          (default) -> errorChecking.movmentError.states.notExpectedToMove.stationary
          errorChecking.movmentError.states.notExpectedToMove.stationary -> errorChecking.movmentError.states.notExpectedToMove.moving : [movingUpOrDown()]
          errorChecking.movmentError.states.notExpectedToMove.moving -> errorChecking.movmentError.states.notExpectedToMove.stationary [order 1] : [!movingUpOrDown()]
        (default) -> (junction 84)
        (junction 84) -> expectedToMove [order 1] : [pwmIn_ex != 0]
        (junction 84) -> (junction 85) [order 2]
        (junction 85) -> expectedToMove [order 1] : [pwmIn_rt != 0]
        (junction 85) -> notExpectedToMove [order 2]
      states -> states [order 2] : [hasChanged(pwmIn_rt)]
      states -> states [order 1] : [hasChanged(pwmIn_ex)]
      (default) -> states
    state positionSensorError [parallel]
      settings: executionOrder=2
      state okay
      state error
        state up
          en,du:
          pwmOut_rt = 0;
          pwmOut_ex = bangBang_maxOut;
        state other
          en,du:
          pwmOut_rt = 0;
          pwmOut_ex = 0;
        state downs
          en,du:
          pwmOut_rt = bangBang_maxOut;
          pwmOut_ex = 0;
        (default) -> (junction 112)
        (junction 112) -> up [order 1] : [targetState == heightUp_e]
        (junction 112) -> (junction 136) [order 2]
        (junction 136) -> (junction 138) [order 1] : [targetState == heightDown_e]
        (junction 136) -> (junction 218) [order 2]
        (junction 138) -> (junction 220)
        (junction 218) -> (junction 220) [order 1] : [targetState == heightMovingDown_e]
        (junction 218) -> other [order 2]
        (junction 220) -> downs
      (default) -> okay
      error -> error [order 2] : [hasChanged(targetState)]
      okay -> error : [legState == heightError_e]
      error -> okay [order 1] : [legState != heightError_e]
  state noChecking
    en,du: pwmOut_ex = pwmIn_ex;
    pwmOut_rt = pwmIn_rt;
  state out = movingUpOrDown [function]
    (default) -> (junction 49)
    (junction 49) -> (junction 51) [order 1] : [legState == heightMovingUp_e]
    (junction 49) -> (junction 53) [order 2]
    (junction 51) -> (junction 55)
    (junction 53) -> (junction 55) [order 1] : [legState == heightMovingDown_e]
    (junction 53) -> (junction 60) [order 2]
    (junction 55) -> (junction 58) : {out = true}
    (junction 60) -> (junction 58) : {out = false}
  state errorWithCommand
    en:
    error.noMovementErr = true;
  state errorWithNoCmdStep1
    en: pwmOut_ex = bangBang_maxOut;
    pwmOut_rt = bangBang_maxOut;
    error.movementErr1 = true;
    state stationary
    state moving
    (default) -> errorWithNoCmdStep1.moving
    errorWithNoCmdStep1.stationary -> errorWithNoCmdStep1.moving : [movingUpOrDown()]
    errorWithNoCmdStep1.moving -> errorWithNoCmdStep1.stationary [order 1] : [!movingUpOrDown()]
  state errorWithNoCmdStep2
    en:
    ccoReqOff = true;
    error.movementErr2 = true;
  errorChecking.movmentError.states.expectedToMove.stationary -> errorWithCommand [order 2] : after(noMovementTimeOut,msec)
  (default) -> errorChecking
  errorChecking -> noChecking [order 1] : [machineState == heightCalibrating_e]
  errorChecking -> noChecking [order 2] : [override]
  (junction 188) -> errorChecking
  errorWithCommand -> (junction 188) : [targetState == heightUnknown_e]
  errorChecking.movmentError.states.notExpectedToMove.moving -> errorWithNoCmdStep1 [order 2] : after(movementTimeOut,msec)
  (junction 214) -> errorChecking : [!override]
  noChecking -> (junction 214) : [machineState != heightCalibrating_e]
  errorWithNoCmdStep1.moving -> errorWithNoCmdStep2 [order 2] : after(movementTimeOut,msec)
  data: out function_output boolean; machineState input; targetState input; legState input; pwmIn_ex input; pwmIn_rt input; pwmOut_ex output single; pwmOut_rt output single; heightDown_e parameter; heightUp_e parameter; heightCalibrating_e parameter; heightError_e parameter; heightUnknown_e parameter; heightMovingDown_e parameter; heightMovingUp_e parameter; bangBang_maxOut parameter; movementTimeOut parameter; noMovementTimeOut parameter; ccoReqOff output boolean =0; error output Bus: ErrorBus =0; override input

== stateflow chart HighClearance_library/trackWidthOkay ==
  state out = trackWidthInTolerance [function]
    (default) -> (junction 35)
    (junction 35) -> (junction 169) [order 1] : [actualTrackPos <= 0]
    (junction 35) -> (junction 174) [order 2]
    (junction 169) -> (junction 176)
    (junction 174) -> (junction 176) [order 1] : [trackCoilErr]
    (junction 174) -> (junction 165) [order 2]
    (junction 176) -> (junction 167)
    (junction 165) -> (junction 40) [order 1] : [(targetTrackPos - actualTrackPos) <= trackWidthTolerance]
    (junction 40) -> (junction 167) : [(actualTrackPos - targetTrackPos) <= trackWidthTolerance]
    (junction 165) -> (junction 42) [order 2] : {out = false}
    (junction 167) -> (junction 41)
    (junction 41) -> (junction 42) : {out = true}
  state checkTolerance
    en,du: enable = trackWidthInTolerance()
  (default) -> checkTolerance
  data: out function_output boolean; targetState input; enable output uint8; targetTrackPos input; actualTrackPos input; trackWidthTolerance parameter; trackCoilErr input boolean

== stateflow chart HighClearance_library/heightOkay ==
  state checkTolerance
    en,du:
    enable_e = heightInTolerance();
  state out = heightInTolerance [function]
    (junction 106) -> (junction 108)
    (junction 117) -> (junction 119)
    (junction 124) -> (junction 128)
    (junction 71) -> (junction 106) [order 1] : [legHeightRef1 == 0]
    (junction 108) -> (junction 122)
    (junction 77) -> (junction 117) [order 1] : [legHeightRef2 == 0]
    (junction 119) -> (junction 125)
    (junction 80) -> (junction 124) [order 1] : [legHeightRef3 == 0]
    (junction 128) -> (junction 81)
    (junction 77) -> (junction 125) [order 2] : [( legHeightSubject - legHeightRef2 ) <= tolerance]
    (junction 125) -> (junction 80)
    (junction 80) -> (junction 81) [order 2] : [( legHeightSubject - legHeightRef3 ) <= tolerance]
    (junction 122) -> (junction 77)
    (junction 71) -> (junction 122) [order 2] : [( legHeightSubject - legHeightRef1 ) <= tolerance]
    (junction 69) -> (junction 71) [order 2] : [targetState == heightUp_e ||...
        | targetState == heightMovingUp_e]
    (junction 77) -> (junction 111) [order 3]
    (junction 80) -> (junction 114) [order 3]
    (junction 81) -> (junction 75) : {out = 1}
    (default) -> (junction 169)
    (junction 169) -> (junction 69) [order 1] : [legHeightSubject != 0]
    (junction 69) -> (junction 111) [order 3]
    (junction 111) -> (junction 114)
    (junction 114) -> (junction 75) : {out = 0}
    (junction 75) -> (junction 177)
    (junction 169) -> (junction 172) [order 2]
    (junction 69) -> (junction 91) [order 1] : [targetState == heightDown_e ||...
        | targetState == heightMovingDown_e]
    (junction 86) -> (junction 111) [order 3]
    (junction 88) -> (junction 114) [order 3]
    (junction 87) -> (junction 75) : {out = 1}
    (junction 173) -> (junction 177) : {out = 3}
    (junction 91) -> (junction 131) [order 1] : [( legHeightRef1 - legHeightSubject ) <= tolerance]
    (junction 131) -> (junction 86)
    (junction 86) -> (junction 132) [order 2] : [( legHeightRef2 - legHeightSubject ) <= tolerance]
    (junction 132) -> (junction 88)
    (junction 88) -> (junction 87) [order 2] : [( legHeightRef3 - legHeightSubject ) <= tolerance]
    (junction 88) -> (junction 151) [order 1] : [legHeightRef3 == 0]
    (junction 91) -> (junction 140) [order 2] : [legHeightRef1 == 0]
    (junction 142) -> (junction 131)
    (junction 86) -> (junction 146) [order 1] : [legHeightRef2 == 0]
    (junction 147) -> (junction 132)
    (junction 153) -> (junction 87)
    (junction 140) -> (junction 142)
    (junction 146) -> (junction 147)
    (junction 151) -> (junction 153)
    (junction 172) -> (junction 173)
  (default) -> checkTolerance
  data: out function_output uint8; targetState input; enable_e output uint8; legHeightSubject input; legHeightRef1 input; legHeightRef2 input; legHeightRef3 input; heightDown_e parameter; heightUp_e parameter; heightMovingUp_e parameter; heightMovingDown_e parameter; heightCalibrating_e parameter; heightError_e parameter; heightUnknown_e parameter; tolerance input

== stateflow chart HighClearance_library/enableLogic ==
  state disabled
    en: enable = false;
    state transitioning
      state okay
      state badTrack
        state wait
        state warning
          en: warningTrack = 1;
          ex: warningTrack = 0;
        (default) -> disabled.transitioning.badTrack.wait
        disabled.transitioning.badTrack.wait -> disabled.transitioning.badTrack.warning : after(ctrlWarningTime,sec)
      state badHeight
        state warning
          en: warningHeight = 1;
          ex: warningHeight = 0;
        state wait
        (default) -> disabled.transitioning.badHeight.wait
        disabled.transitioning.badHeight.wait -> disabled.transitioning.badHeight.warning : after(ctrlWarningTime,sec)
      (default) -> okay
      okay -> badTrack [order 1] : [!trackWidthInTolerance]
      badTrack -> okay : [trackWidthInTolerance]
      okay -> badHeight [order 2] : [heightInTolerance == 0]
      badHeight -> okay : [heightInTolerance != 0]
    state NotTransitioning
      en:
      warningTrack = 0;
      warningHeight = 0;
    (default) -> NotTransitioning
    NotTransitioning -> transitioning [order 1] : [targetState == heightMovingUp_e]
    NotTransitioning -> transitioning [order 2] : [targetState == heightMovingDown_e]
    (junction 183) -> NotTransitioning : [targetState != heightMovingUp_e]
    transitioning -> (junction 183) : [targetState != heightMovingDown_e]
  state enabled
    en: enable = true;
  (default) -> disabled
  disabled -> (junction 38) : [trackWidthInTolerance]
  (junction 38) -> enabled : [heightInTolerance == 1]
  enabled -> disabled [order 2] : [!trackWidthInTolerance]
  enabled -> disabled [order 1] : [heightInTolerance != 1]
  data: targetState input; enable output uint8; heightDown_e parameter; heightUp_e parameter; heightMovingUp_e parameter; heightMovingDown_e parameter; heightCalibrating_e parameter; heightError_e parameter; heightUnknown_e parameter; trackWidthTolerance parameter; heightDiffTolerance parameter; warningTrack output uint8; warningHeight output uint8; trackWidthInTolerance input; heightInTolerance input; ctrlWarningTime parameter
